simulink model "untitled2"  (R2016a)
settings: Solver=VariableStepAuto  StartTime=0.0  StopTime=10.0  RelTol=1e-3
settings Model: Creator=Utilizator  LastModifiedBy=Utilizator

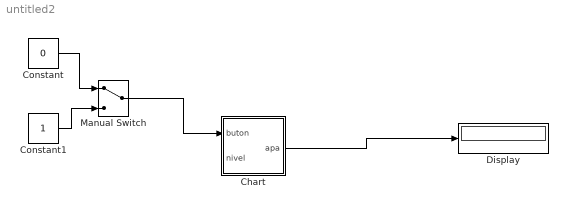
== system untitled2 ==
  Chart : Stateflow chart  TreatAsAtomicUnit=on
  Constant : Constant  Value=0
  Constant1 : Constant
  Display : Display
  Manual Switch : ManualSwitch
  wires:
  Constant/1 -> Manual Switch/1
  Constant1/1 -> Manual Switch/2
  Manual Switch/1 -> Chart/1(buton)
  Chart/1(apa) -> Display/1

== stateflow chart untitled2/Chart ==
  state ON
    entry: apa=1;
    int=0;
    dialog ctr = ctr + 1;
  state OFF
    entry: apa=0;
    ctr=0;
  state ONBazin
  state OFFBazin
  OFF -> ON [order 1] : [buton==1 || int==1]
  (default) -> OFF
  OFFBazin -> OFF
  ON -> OFF [order 1] : [buton==0 && ctr==10]
  OFF -> ONBazin [order 2] : [buton==1]
  ON -> ONBazin [order 2] : [nivel==1]
  ONBazin -> OFFBazin : [nivel==1]
  data: buton input; apa output; ctr local; int local =1; nivel input
